simulink model "motor"  (Simulink 7.8)
settings: Solver=ode3  StartTime=0.0  StopTime=1  FixedStep=Ts  RelTol=1e-3
PostLoadFcn:
  | Ts=1e-6;Fc=1e4;
InitFcn:
  | Ts=1e-6;Fc=1e4;
libraries: powerlib x7, simulink x3
settings Model: Creator=Administrator  LastModifiedBy=Administrator

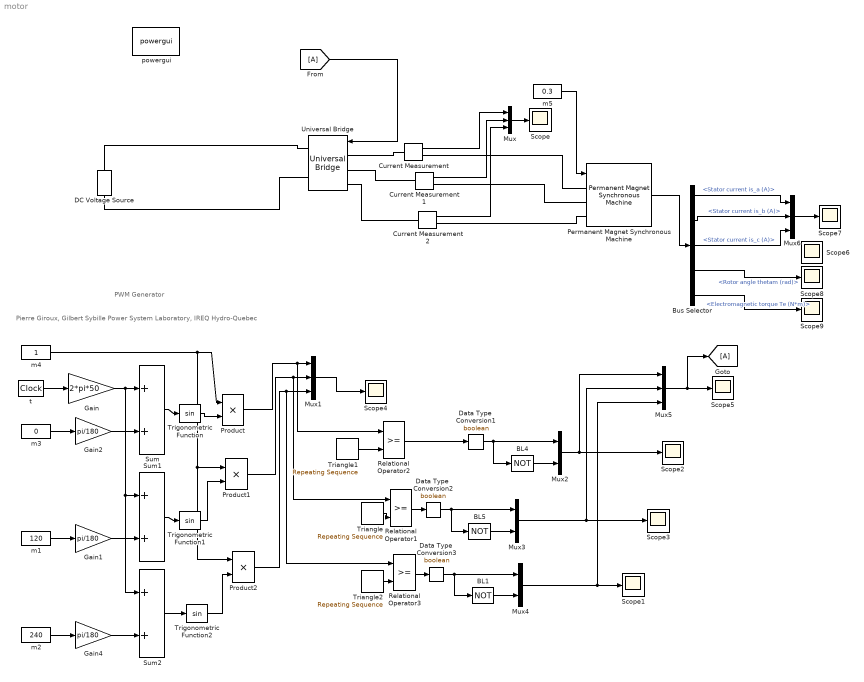
== system motor ==
  note: Pierre Giroux, Gilbert Sybille
      | Power System Laboratory, IREQ
      | Hydro-Quebec
  note: PWM Generator
  BL1 : Logic  Operator=NOT  Inputs=1  SampleTime=Ts
  BL4 : Logic  Operator=NOT  Inputs=1  SampleTime=Ts
  BL5 : Logic  Operator=NOT  Inputs=1  SampleTime=Ts
  Bus Selector : BusSelector  OutputSignals=Stator current is_a (A),Stator current is_b (A),Stator current is_c (A),Rotor angle thetam (rad),Electromagnetic torque Te (N*m)
  Current Measurement : powerlib/Measurements/Current Measurement  PhasorSimulation=off  OutputType=Complex  PSBequivalent=0
  Current Measurement1 : powerlib/Measurements/Current Measurement  PhasorSimulation=off  OutputType=Complex  PSBequivalent=0
  Current Measurement2 : powerlib/Measurements/Current Measurement  PhasorSimulation=off  OutputType=Complex  PSBequivalent=0
  DC Voltage Source : powerlib/Electrical Sources/DC Voltage Source  Amplitude=350  Measurements=None
  Data Type  Conversion1 : DataTypeConversion  OutDataTypeStr=boolean  SampleTime=Ts  SaturateOnIntegerOverflow=on  RndMeth=Zero
  Data Type  Conversion2 : DataTypeConversion  OutDataTypeStr=boolean  SampleTime=Ts  SaturateOnIntegerOverflow=on  RndMeth=Zero
  Data Type  Conversion3 : DataTypeConversion  OutDataTypeStr=boolean  SampleTime=Ts  SaturateOnIntegerOverflow=on  RndMeth=Zero
  Gain : Gain  Gain=2*pi*50  SaturateOnIntegerOverflow=on  OutDataTypeStr=Inherit: Same as input  ParamDataTypeStr=Inherit: Same as input
  Gain1 : Gain  Gain=pi/180  SaturateOnIntegerOverflow=on  OutDataTypeStr=Inherit: Same as input  ParamDataTypeStr=Inherit: Same as input
  Gain2 : Gain  Gain=pi/180  SaturateOnIntegerOverflow=on  OutDataTypeStr=Inherit: Same as input  ParamDataTypeStr=Inherit: Same as input
  Gain4 : Gain  Gain=pi/180  SaturateOnIntegerOverflow=on  OutDataTypeStr=Inherit: Same as input  ParamDataTypeStr=Inherit: Same as input
  Mux{,1,5..6} (4 alike) : Mux  Inputs=3
  Mux2 : Mux  Inputs=2
  Mux3 : Mux  Inputs=2
  Mux4 : Mux  Inputs=2
  Permanent Magnet Synchronous Machine : powerlib/Machines/Permanent Magnet Synchronous Machine  NbPhases=3  FluxDistribution=Sinusoidal  RotorType=Round  MechanicalLoad=Torque Tm  PresetModel="08:  24 Nm 300 Vdc 2300 RPM - 41.4 Nm"  ShowDetailedParameters=on  Resistance=0.0918  Inductance=8.5e-3  dqInductances=[8.5e-3,8.5e-3]  La=0.000975  MachineConstant=Flux linkage established by magnets (V.s)  Flux=0.1688  VoltageCst=51.8384  TorqueCst=0.4287  Flat=120  Mechanical=[0.003945 0.0004924 4 0]  PolePairs=4  InitialConditions=[0,0, 0,0]  InitialConditions5ph=[0 0 0 0 0 0]  TsPowergui=0  TsBlock=-1  RefAngle=90 degrees behind phase A axis (modified Park)
  Product : Product  SampleTime=Ts  SaturateOnIntegerOverflow=on  InputSameDT=on  OutDataTypeStr=Inherit: Same as first input
  Product1 : Product  SampleTime=Ts  SaturateOnIntegerOverflow=on  InputSameDT=on  OutDataTypeStr=Inherit: Same as first input
  Product2 : Product  SampleTime=Ts  SaturateOnIntegerOverflow=on  InputSameDT=on  OutDataTypeStr=Inherit: Same as first input
  Relational Operator1 : RelationalOperator  SampleTime=Ts  InputSameDT=on
  Relational Operator2 : RelationalOperator  SampleTime=Ts  InputSameDT=on
  Relational Operator3 : RelationalOperator  SampleTime=Ts  InputSameDT=on
  Scope{,1..9} (10 alike) : Scope
      Scope settings: YMin=-7.5  YMax=7.5
      Scope2 settings: SaveName=ScopeData2
      Scope3 settings: SaveName=ScopeData3
      Scope4 settings: SaveName=ScopeData4
      Scope5 settings: SaveName=ScopeData5
      Scope6 settings: SaveName=ScopeData6
      Scope7 settings: YMin=-500  YMax=550  SaveName=ScopeData7
      Scope8 settings: SaveName=ScopeData8
      Scope9 settings: SaveName=ScopeData9
  Sum : Sum  SampleTime=Ts  SaturateOnIntegerOverflow=on  InputSameDT=on  OutDataTypeStr=Inherit: Same as first input
  Sum1 : Sum  SampleTime=Ts  SaturateOnIntegerOverflow=on  InputSameDT=on  OutDataTypeStr=Inherit: Same as first input
  Sum2 : Sum  SampleTime=Ts  SaturateOnIntegerOverflow=on  InputSameDT=on  OutDataTypeStr=Inherit: Same as first input
  Triangle : simulink/Sources/Repeating Sequence  rep_seq_t=[0 1/Fc/4 3/Fc/4 1/Fc]  rep_seq_y=[0 -1 1 0]
  Triangle1 : simulink/Sources/Repeating Sequence  rep_seq_t=[0 1/Fc/4 3/Fc/4 1/Fc]  rep_seq_y=[0 -1 1 0]
  Triangle2 : simulink/Sources/Repeating Sequence  rep_seq_t=[0 1/Fc/4 3/Fc/4 1/Fc]  rep_seq_y=[0 -1 1 0]
  Trigonometric Function : Trigonometry  SampleTime=Ts
  Trigonometric Function1 : Trigonometry  SampleTime=Ts
  Trigonometric Function2 : Trigonometry  SampleTime=Ts
  Universal Bridge : powerlib/Power Electronics/Universal Bridge  Arms=3  SnubberResistance=1e5  SnubberCapacitance=inf  Device=IGBT / Diodes  Ron=1e-3  Lon=0  ForwardVoltages="[  0  0  ]"  ForwardVoltage=0  GTOparameters=[ 10e-6 , 20e-6 ]  IGBTparameters=[ 1e-6 , 2e-6 ]  Measurements=None  Measurements_2=None  converterType=Rectifier
  m1 : Constant  Value=120  SampleTime=Ts
  m2 : Constant  Value=240  SampleTime=Ts
  m3 : Constant  Value=0  SampleTime=Ts
  m4 : Constant  SampleTime=Ts
  m5 : Constant  Value=0.3  SampleTime=Ts
  powergui : powerlib/powergui  Priority=1  SimulationMode=Continuous  SolverType=Tustin  SampleTime=50e-6  frequency=60  SPID=off  DisableSnubberDevices=off  DisableRonSwitches=off  DisableVfSwitches=off  SwTol=0  Interpol=off  DisplayEquations=off  FunctionMessages=off  frequencyindice=0  Pbase=100e6  ErrMax=1e-4  Iterations=50  UnitsV=kV  UnitsW=MW  echomessages=off  HookPort=off  EnableUseOfTLC=off  x0status=blocks  RestoreLinks=warning  ResistiveCurrentMeasurement=off  Ylog=off  Xlog=on  ShowGrid=off  save=off  variable=ZData  ZoomFFT=off  StartTime=0.0  cycles=1  DisplayStyle=1  FreqAxis=off  MaxFrequency=1000  frequencyindicesteady=1  display=off  methode=off
  t : DigitalClock  SampleTime=Ts
  wires:
  Current Measurement/1 -> Mux/1
  Current Measurement1/1 -> Mux/2
  Current Measurement2/1 -> Mux/3
  Mux/1 -> Scope/1
  [A] -> Universal Bridge/1
  Mux3/1 -> Scope3/1, Mux5/2
  Mux2/1 -> Scope2/1, Mux5/1
  BL5/1 -> Mux3/2
  BL4/1 -> Mux2/2
  Triangle/1 -> Relational Operator1/2
  Trigonometric Function/1 -> Product/2
  Sum/1 -> Trigonometric Function/1
  m4/1 -> Product/1, Product1/1, Product2/1
  m3/1 -> Gain2/1
  Gain2/1 -> Sum/2
  Gain/1 -> Sum/1, Sum1/1, Sum2/1
  t/1 -> Gain/1
  Relational Operator2/1 -> Data Type  Conversion1/1
  Data Type  Conversion1/1 -> BL4/1, Mux2/1
  Relational Operator1/1 -> Data Type  Conversion2/1
  Data Type  Conversion2/1 -> BL5/1, Mux3/1
  Sum1/1 -> Trigonometric Function1/1
  Trigonometric Function1/1 -> Product1/2
  m1/1 -> Gain1/1
  Gain1/1 -> Sum1/2
  m2/1 -> Gain4/1
  Gain4/1 -> Sum2/2
  Trigonometric Function2/1 -> Product2/2
  Sum2/1 -> Trigonometric Function2/1
  Product/1 -> Mux1/1, Relational Operator2/1
  Product1/1 -> Mux1/2, Relational Operator1/1
  Product2/1 -> Mux1/3, Relational Operator3/1
  Mux1/1 -> Scope4/1
  Triangle1/1 -> Relational Operator2/2
  Mux4/1 -> Scope1/1, Mux5/3
  BL1/1 -> Mux4/2
  Triangle2/1 -> Relational Operator3/2
  Relational Operator3/1 -> Data Type  Conversion3/1
  Data Type  Conversion3/1 -> Mux4/1, BL1/1
  Mux5/1 -> Scope5/1, [A]
  Permanent Magnet Synchronous Machine/1 -> Bus Selector/1
  Mux6/1 -> Scope7/1
  Bus Selector/1 -> Mux6/1  "<Stator current is_a (A)>"
  Bus Selector/2 -> Mux6/2  "<Stator current is_b (A)>"
  Bus Selector/3 -> Mux6/3  "<Stator current is_c (A)>"
  ? -> Scope6/1  "<s)>"
  Bus Selector/4 -> Scope8/1  "<Rotor angle thetam (rad)>"
  Bus Selector/5 -> Scope9/1  "<Electromagnetic torque Te (N*m)>"
  m5/1 -> Permanent Magnet Synchronous Machine/1
  connections:
  DC Voltage Source/RConn1 -- Universal Bridge/RConn1
  DC Voltage Source/LConn1 -- Universal Bridge/RConn2
  Current Measurement/LConn1 -- Universal Bridge/LConn1
  Current Measurement1/LConn1 -- Universal Bridge/LConn2
  Current Measurement2/LConn1 -- Universal Bridge/LConn3
  Current Measurement1/RConn1 -- Permanent Magnet Synchronous Machine/LConn2
  Current Measurement2/RConn1 -- Permanent Magnet Synchronous Machine/LConn3
  Current Measurement/RConn1 -- Permanent Magnet Synchronous Machine/LConn1
